simulink model "robot_v3_m1"  (R2022b)
settings: Solver=FixedStepDiscrete  StartTime=0.0  StopTime=10.0  FixedStep=T_S  RelTol=1e-3  EnableMultiTasking=on
values from neighbouring files (symbols this model uses):
  T_S = 10e-3    (= 0.01)    [robot_prototype_init.m]
undefined symbols (not defined in the file or in its folder): Break, Btn, btn, Button, Ctr, State, Up
libraries: legoev3lib x23
settings Model: ExtModeTrigDuration=2  Creator=hp  LastModifiedBy=hp
settings SolverCC: PositivePriorityOrder=on
settings OptimizationCC: EnhancedBackFolding=on  PassReuseOutputArgsAs=Individual arguments  ZeroExternalMemoryAtStartup=off  ZeroInternalMemoryAtStartup=off  MaxStackSize=64  OptimizeBlockOrder=speed  DifferentSizesBufferReuse=on  OptimizationCustomize=off  EfficientTunableParamExpr=on
settings DebuggingCC: ParameterTunabilityLossMsg=error
settings HardwareCC: ProdBitPerPointer=32  ProdBitPerSizeT=32  ProdBitPerPtrDiffT=32  ProdLargestAtomicInteger=Long  ProdWordSize=32  ProdHWDeviceType=ARM Compatible->ARM 9
settings SFSimCC: MATLABDynamicMemAlloc=off
settings RTWCC: Description=Embedded Coder  SystemTargetFile=ert.tlc  HardwareBoard=LEGO MINDSTORMS EV3  TLCOptions="-aInlineSetEventsForThisBaseRateFcn=TLC_FALSE -aSuppressMultiTaskScheduler=TLC_FALSE  -aRateBasedStepFcn=0"  TemplateMakefile=ert_default_tmf  Toolchain=Sourcery G++ Lite v2009q3
settings CodeAppCC: ForceParamTrailComments=on  IgnoreCustomStorageClasses=off  OperatorAnnotations=on  SimulinkDataObjDesc=on  SFDataObjDesc=on  InsertBlockDesc=on
settings ERTTargetCC: SupportContinuousTime=on  SupportVariableSizeSignals=on  ExtModeTransport=2  ExtModeStaticAlloc=on  ExtModeMexFile=ext_xcp  ExtModeIntrfLevel=Level2 - Open

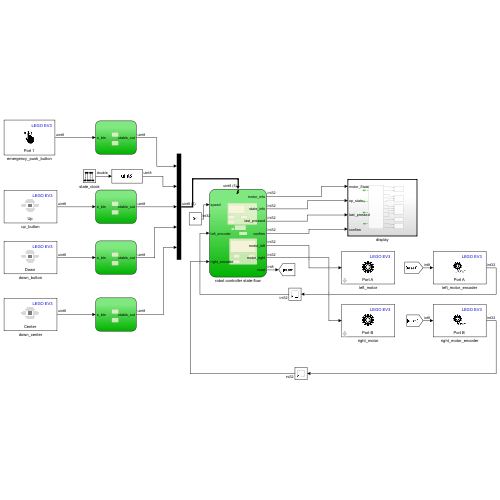
[thumbnail: Simulink's stored preview of the top-level diagram]
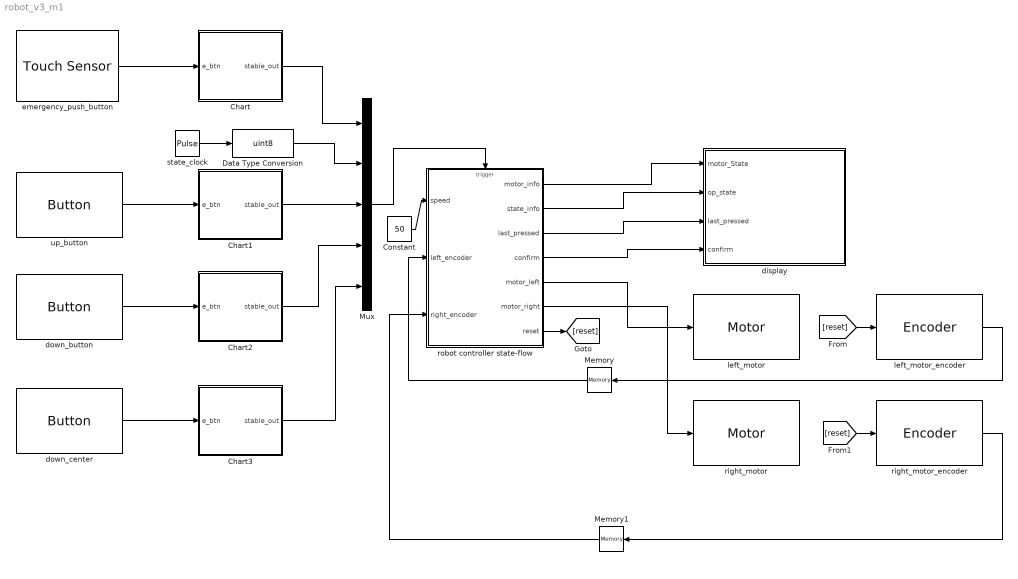
== system robot_v3_m1 ==
  Chart : Stateflow chart  TreatAsAtomicUnit=on
  Chart1 : Stateflow chart  TreatAsAtomicUnit=on
  Chart2 : Stateflow chart  TreatAsAtomicUnit=on
  Chart3 : Stateflow chart  TreatAsAtomicUnit=on
  Constant : Constant  Value=50  OutDataTypeStr=int32
  Data Type Conversion : DataTypeConversion  OutMin=0  OutMax=255  OutDataTypeStr=uint8  SaturateOnIntegerOverflow=off  RndMeth=Floor
  Memory : Memory
  Memory1 : Memory
  Mux : Mux  Inputs=5
  display : Subsystem  TreatAsAtomicUnit=on
  down_button : legoev3lib/Button  buttonType=Down  sampleTime=T_S
  down_center : legoev3lib/Button  buttonType=Center  sampleTime=T_S
  emergency_push_button : legoev3lib/Touch Sensor  portNumber=1  sampleTime=T_S
  left_motor : legoev3lib/Motor  sportNumber=A  sstopAction=Brake
  left_motor_encoder : legoev3lib/Encoder  portNumber=A  opMode=Reset by external signal  sampleTime=T_S
  right_motor : legoev3lib/Motor  sportNumber=B  sstopAction=Brake
  right_motor_encoder : legoev3lib/Encoder  portNumber=B  opMode=Reset by external signal  sampleTime=T_S
  robot controller state-flow : Stateflow chart  TreatAsAtomicUnit=on
  state_clock : DiscretePulseGenerator  Period=50  PulseWidth=25  PhaseDelay=20  SampleTime=T_S
  up_button : legoev3lib/Button  buttonType=Up  sampleTime=T_S
  wires:
  emergency_push_button/1 -> Chart/1(e_btn)
  robot controller state-flow/2(state_info) -> display/2(op_state)
  robot controller state-flow/1(motor_info) -> display/1(motor_State)
  Chart1/1(stable_out) -> Mux/3
  robot controller state-flow/4(confirm) -> display/4(confirm)
  robot controller state-flow/3(last_pressed) -> display/3(last_pressed)
  Chart3/1(stable_out) -> Mux/5
  up_button/1 -> Chart1/1(e_btn)
  Chart/1(stable_out) -> Mux/1
  Data Type Conversion/1 -> Mux/2
  Mux/1 -> robot controller state-flow/Trigger
  state_clock/1 -> Data Type Conversion/1
  down_button/1 -> Chart2/1(e_btn)
  Constant/1 -> robot controller state-flow/1(speed)
  down_center/1 -> Chart3/1(e_btn)
  Chart2/1(stable_out) -> Mux/4
  [reset] -> left_motor_encoder/1
  [reset] -> right_motor_encoder/1
  robot controller state-flow/5(motor_left) -> left_motor/1
  robot controller state-flow/6(motor_right) -> right_motor/1
  robot controller state-flow/7(reset) -> [reset]
  left_motor_encoder/1 -> Memory/1
  right_motor_encoder/1 -> Memory1/1
  Memory/1 -> robot controller state-flow/2(left_encoder)
  Memory1/1 -> robot controller state-flow/3(right_encoder)

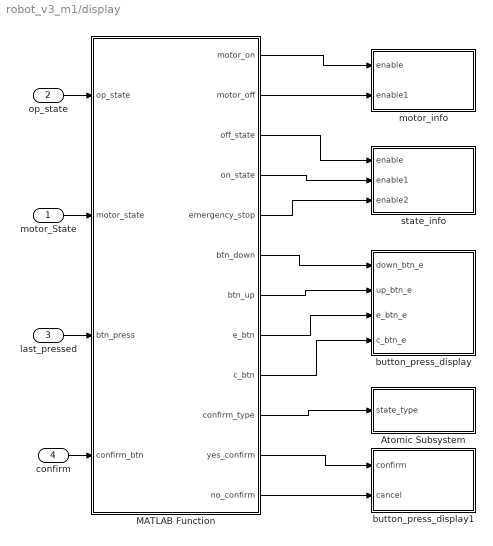
== system robot_v3_m1/display ==
  motor_State : Inport
  op_state : Inport  Port=2
  last_pressed : Inport  Port=3
  confirm : Inport  Port=4
  Atomic Subsystem : Subsystem
  MATLAB Function : MATLAB Function  TreatAsAtomicUnit=on
  button_press_display : Subsystem  SystemSampleTime=T_S
  button_press_display1 : Subsystem  SystemSampleTime=T_S
  motor_info : Subsystem  SystemSampleTime=T_S
  state_info : Subsystem  SystemSampleTime=T_S
  wires:
  op_state/1 -> MATLAB Function/1(op_state)
  motor_State/1 -> MATLAB Function/2(motor_state)
  MATLAB Function/3(off_state) -> state_info/1(enable)
  MATLAB Function/4(on_state) -> state_info/2(enable1)
  MATLAB Function/5(emergency_stop) -> state_info/3(enable2)
  MATLAB Function/1(motor_on) -> motor_info/1(enable)
  MATLAB Function/2(motor_off) -> motor_info/2(enable1)
  last_pressed/1 -> MATLAB Function/3(btn_press)
  MATLAB Function/6(btn_down) -> button_press_display/1(down_btn_e)
  MATLAB Function/7(btn_up) -> button_press_display/2(up_btn_e)
  MATLAB Function/8(e_btn) -> button_press_display/3(e_btn_e)
  confirm/1 -> MATLAB Function/4(confirm_btn)
  MATLAB Function/10(confirm_type) -> Atomic Subsystem/1(state_type)
  MATLAB Function/11(yes_confirm) -> button_press_display1/1(confirm)
  MATLAB Function/12(no_confirm) -> button_press_display1/2(cancel)
  MATLAB Function/9(c_btn) -> button_press_display/4(c_btn_e)

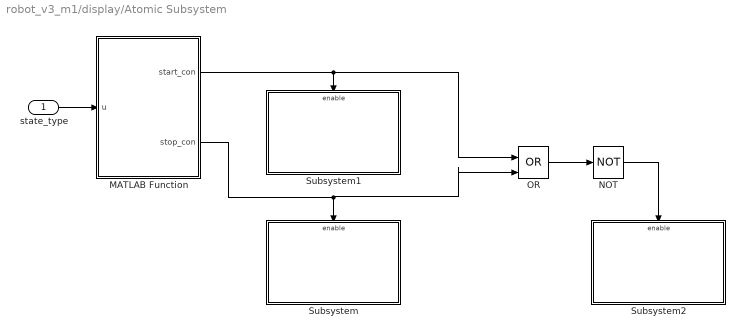
== system robot_v3_m1/display/Atomic Subsystem ==
  state_type : Inport
  MATLAB Function : MATLAB Function  TreatAsAtomicUnit=on
  NOT : Logic  Operator=NOT  IconShape=distinctive  AllPortsSameDT=off  OutDataTypeStr=boolean
  OR : Logic  Operator=OR  IconShape=distinctive  AllPortsSameDT=off  OutDataTypeStr=boolean
  Subsystem : Subsystem
  Subsystem1 : Subsystem
  Subsystem2 : Subsystem
  wires:
  state_type/1 -> MATLAB Function/1(u)
  MATLAB Function/1(start_con) -> OR/1, Subsystem1/Enable
  NOT/1 -> Subsystem2/Enable
  MATLAB Function/2(stop_con) -> OR/2, Subsystem/Enable
  OR/1 -> NOT/1

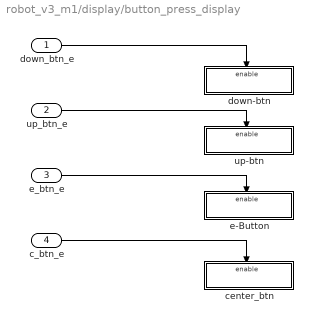
== system robot_v3_m1/display/button_press_display ==
  down_btn_e : Inport
  up_btn_e : Inport  Port=2
  e_btn_e : Inport  Port=3
  c_btn_e : Inport  Port=4
  center_btn : Subsystem
  down-btn : Subsystem
  e-Button : Subsystem
  up-btn : Subsystem
  wires:
  up_btn_e/1 -> up-btn/Enable
  down_btn_e/1 -> down-btn/Enable
  e_btn_e/1 -> e-Button/Enable
  c_btn_e/1 -> center_btn/Enable

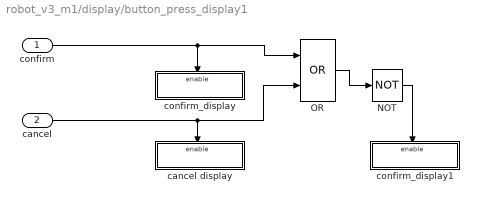
== system robot_v3_m1/display/button_press_display1 ==
  confirm : Inport
  cancel : Inport  Port=2
  NOT : Logic  Operator=NOT  IconShape=distinctive  AllPortsSameDT=off  OutDataTypeStr=boolean
  OR : Logic  Operator=OR  IconShape=distinctive  AllPortsSameDT=off  OutDataTypeStr=boolean
  cancel display : Subsystem
  confirm_display : Subsystem
  confirm_display1 : Subsystem
  wires:
  confirm/1 -> OR/1, confirm_display/Enable
  cancel/1 -> cancel display/Enable, OR/2
  OR/1 -> NOT/1
  NOT/1 -> confirm_display1/Enable

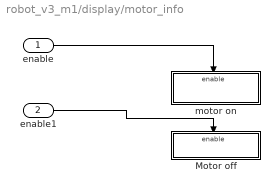
== system robot_v3_m1/display/motor_info ==
  enable : Inport
  enable1 : Inport  Port=2
  Motor off : Subsystem
  motor on : Subsystem
  wires:
  enable/1 -> motor on/Enable
  enable1/1 -> Motor off/Enable

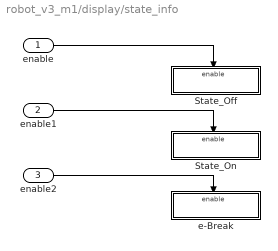
== system robot_v3_m1/display/state_info ==
  enable : Inport
  enable1 : Inport  Port=2
  enable2 : Inport  Port=3
  State_Off : Subsystem
  State_On : Subsystem
  e-Break : Subsystem
  wires:
  enable/1 -> State_Off/Enable
  enable2/1 -> e-Break/Enable
  enable1/1 -> State_On/Enable

== system robot_v3_m1/display/Atomic Subsystem/Subsystem ==
  Enable : EnablePort  StatesWhenEnabling=reset
  stop_confirm : legoev3lib/Display  slcdStr=STOP?  slcdLine=4  slcdFormat=Decimal

== system robot_v3_m1/display/Atomic Subsystem/Subsystem1 ==
  Enable : EnablePort  StatesWhenEnabling=reset
  start_confirm : legoev3lib/Display  slcdStr=START?  slcdLine=4  slcdFormat=Decimal

== system robot_v3_m1/display/Atomic Subsystem/Subsystem2 ==
  Enable : EnablePort  StatesWhenEnabling=reset
  start_confirm : legoev3lib/Display  slcdStr=>>  slcdLine=4  slcdFormat=Decimal

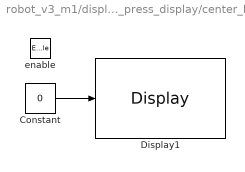
== system robot_v3_m1/display/button_press_display/center_btn ==
  enable : EnablePort  StatesWhenEnabling=reset
  Constant : Constant  Value=0
  Display1 : legoev3lib/Display  slcdStr=Ctr-Btn  slcdLine=10  slcdFormat=Hex
  wires:
  Constant/1 -> Display1/1

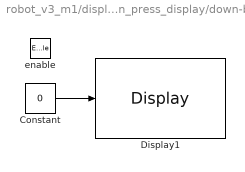
== system robot_v3_m1/display/button_press_display/down-btn ==
  enable : EnablePort  StatesWhenEnabling=reset
  Constant : Constant  Value=0
  Display1 : legoev3lib/Display  slcdStr=btn-down  slcdLine=10  slcdFormat=Hex
  wires:
  Constant/1 -> Display1/1

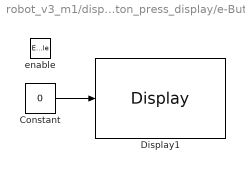
== system robot_v3_m1/display/button_press_display/e-Button ==
  enable : EnablePort  StatesWhenEnabling=reset
  Constant : Constant  Value=0
  Display1 : legoev3lib/Display  slcdStr=E-Button  slcdLine=10  slcdFormat=Hex
  wires:
  Constant/1 -> Display1/1

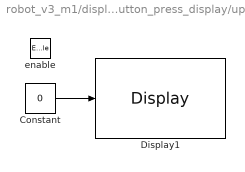
== system robot_v3_m1/display/button_press_display/up-btn ==
  enable : EnablePort  StatesWhenEnabling=reset
  Constant : Constant  Value=0
  Display1 : legoev3lib/Display  slcdStr=btn-Up  slcdLine=10  slcdFormat=Hex
  wires:
  Constant/1 -> Display1/1

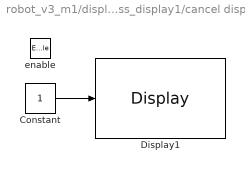
== system robot_v3_m1/display/button_press_display1/cancel display ==
  enable : EnablePort  StatesWhenEnabling=reset
  Constant : Constant
  Display1 : legoev3lib/Display  slcdStr=Cancel  slcdLine=5  slcdFormat=Hex
  wires:
  Constant/1 -> Display1/1

== system robot_v3_m1/display/button_press_display1/confirm_display ==
  enable : EnablePort  StatesWhenEnabling=reset
  Constant : Constant
  Display1 : legoev3lib/Display  slcdStr=Confrim  slcdLine=5  slcdFormat=Hex
  wires:
  Constant/1 -> Display1/1

== system robot_v3_m1/display/button_press_display1/confirm_display1 ==
  enable : EnablePort  StatesWhenEnabling=reset
  Display1 : legoev3lib/Display  slcdStr=>>  slcdLine=5  slcdFormat=Hex

== system robot_v3_m1/display/motor_info/Motor off ==
  enable : EnablePort  StatesWhenEnabling=reset
  Constant : Constant  Value=0
  Display1 : legoev3lib/Display  slcdStr=motorOff  slcdLine=2  slcdFormat=Hex
  wires:
  Constant/1 -> Display1/1

== system robot_v3_m1/display/motor_info/motor on ==
  enable : EnablePort  StatesWhenEnabling=reset
  Constant : Constant  Value=0  SampleTime=T_S
  Display1 : legoev3lib/Display  slcdStr=motorOn  slcdLine=2  slcdFormat=Hex
  wires:
  Constant/1 -> Display1/1

== system robot_v3_m1/display/state_info/State_Off ==
  enable : EnablePort  StatesWhenEnabling=reset
  Constant : Constant  Value=0
  Display1 : legoev3lib/Display  slcdStr=StateOff  slcdLine=1  slcdFormat=Hex
  wires:
  Constant/1 -> Display1/1

== system robot_v3_m1/display/state_info/State_On ==
  enable : EnablePort  StatesWhenEnabling=reset
  Constant : Constant  Value=0
  Display1 : legoev3lib/Display  slcdStr=State-On  slcdLine=1  slcdFormat=Hex
  wires:
  Constant/1 -> Display1/1

== system robot_v3_m1/display/state_info/e-Break ==
  enable : EnablePort  StatesWhenEnabling=reset
  Constant : Constant  Value=0
  Display1 : legoev3lib/Display  slcdStr=E-Break  slcdLine=1  slcdFormat=Hex
  wires:
  Constant/1 -> Display1/1

== stateflow chart robot_v3_m1/Chart ==
  state off
    entry:
    stable_out = 0
  note: ]
  state on
    entry:
    stable_out = 1
  (default) -> off
  on -> off : [duration(e_btn<0.3) > 20e-3]
  off -> on : [duration(e_btn> 0.7) > 20e-3]
  data: e_btn input; stable_out output uint8

== matlab function robot_v3_m1/display/MATLAB Function ==
  data: op_state input; motor_on output; motor_off output; motor_state input; off_state output; on_state output; emergency_stop output; btn_down output; btn_up output; e_btn output; c_btn output; btn_press input; confirm_btn input; confirm_type output; yes_confirm output; no_confirm output
function [motor_on,motor_off, off_state, on_state, emergency_stop, btn_down, btn_up ,e_btn, c_btn , confirm_type ,yes_confirm, no_confirm] = fcn(op_state, motor_state, btn_press, confirm_btn)

motor_on = 0;
motor_off = 0;

off_state = 0;
on_state = 0;
emergency_stop = 0;

btn_down = 0;
btn_up = 0;
e_btn = 0;
c_btn = 0;

confirm_type = 0;
yes_confirm = 0;
no_confirm = 0;

% for displaying motor state
if motor_state == 0
    motor_off = 1;
elseif motor_state == 1
    motor_on = 1;
end

% for displaying states
if op_state == 0
    off_state = 1;
elseif op_state == 1
    on_state = 1;
elseif op_state == 2
    emergency_stop = 1;
end

%for displaying button press
if btn_press == 1
    btn_down = 1;
elseif btn_press == 2
    btn_up = 1;
elseif btn_press == 3
    e_btn = 1;
elseif btn_press == 4
    c_btn = 1;
end

%for displaying which action to confirm
%i.e. either star action or stop action
if confirm_btn == 1 | confirm_btn == 2
    confirm_type = 1;
elseif confirm_btn == 3 | confirm_btn == 4
    confirm_type = 2;
end

if confirm_btn == 1 && confirm_type == 1
    yes_confirm = 1;
elseif confirm_btn == 2 && confirm_type == 1
    no_confirm = 1;
end

if confirm_btn == 3 && confirm_type == 2
    yes_confirm = 1;
elseif confirm_btn == 4 && confirm_type == 2
    no_confirm = 1;
end

== stateflow chart robot_v3_m1/robot controller state-flow ==
  state Off_super_state
    entry:
    state state_off
      entry:
      motor_left = 0;
      motor_right = 0;
      motor_info = 0;
      state_info = 0;
      confirm = 0;
      e_press_count = 0;
      last_pressed = button_type;
      stop_robot = int32(0);
    state confirm_start_action_
      entry:
      confirm = 1;
      last_pressed = button_type;
    state cancel_start_action
      entry:
      confirm = 2;
      last_pressed = button_type;
    state confirmed_start
      entry:
      start_robot = 1;
      last_pressed = button_type;
      confirm = 0;
    (default) -> state_off
    state_off -> confirm_start_action_ : up_btn{button_type = 2}
    cancel_start_action -> state_off [order 1] : center_btn{confirm = 0;
        | button_type = 4;}
    cancel_start_action -> confirm_start_action_ [order 2] : up_btn{button_type = 2;}
    confirm_start_action_ -> cancel_start_action [order 2] : down_btn{button_type = 1}
    confirm_start_action_ -> confirmed_start [order 1] : center_btn{
        | button_type = 4}
  note: button_type is internal variable used to store which button was pressed
      | 0 = no button press
      | 1 = down
      | 2 = up
      | 3 = emergency_button
      | 4 = center_button
  note: These confirmation applies when confirming to turn on the robot
      |
      | confirm = 1
      | display 1 at the confirm position
      | confirm = 2
      | display 1 at cancel position
      |
      | 0
      | anything else don't display anything.
  state emergency_stop
    entry:
    motor_left = 0;
    motor_right = 0;
    motor_info = 0;
    state_info = 2;
    last_pressed = button_type;
  note: state_info
      | 0 = off_state
      | 1 = Turned on
      | 2 = emergency top
  state leyway
    entry:
    reset = 0;
  state intermediate
    entry:
    e_press_count = e_press_count +1;
  state go
    entry:
    state action
      entry:
      motor_info = 1;
      state_info = 1;
      last_pressed = button_type;
      start_robot = int32(0);
      e_press_count = int32(0);
      during:
      if (2046 - left_encoder) >0
      motor_left  =  speed;
      else
      motor_left = 0;
      end
      if (2046 - right_encoder) >0
      motor_right  =  speed;
      else
      motor_right = 0;
      end
      exit:
      motor_left = 0;
      motor_right = 0;
    state confirm_stop_action
      entry:
      confirm = 3;
      motor_info = 0;
      last_pressed = button_type;
    state cancel_stop_action
      entry:
      confirm = 4;
      last_pressed = button_type;
    state confirmed_stop
      entry:
      stop_robot = 1;
      last_pressed = button_type;
      confirm = 0;
      exit:
      reset = 1;
    (default) -> action
    action -> confirm_stop_action : down_btn{button_type = 1}
    cancel_stop_action -> action [order 1] : center_btn{confirm = 0;
        | button_type = 4;}
    cancel_stop_action -> confirm_stop_action [order 2] : up_btn{button_type = 2;}
    confirm_stop_action -> cancel_stop_action [order 2] : down_btn{button_type = 1}
    confirm_stop_action -> confirmed_stop [order 1] : center_btn{
        | button_type = 4}
  (default) -> Off_super_state
  go -> Off_super_state [order 2] : [stop_robot == 1]{confirm = 0; button_type = 1;}
  Off_super_state -> leyway : [start_robot == 1]{button_type = 4;confirm = 0;}
  go -> emergency_stop [order 1] : emergency_btn{
      | button_type = 3}
  emergency_stop -> go [order 2] : [e_press_count == 2]
  emergency_stop -> intermediate [order 1] : emergency_btn
  intermediate -> emergency_stop [order 1] : after(0.5, sec){e_press_count = 0;}
  intermediate -> emergency_stop [order 2] : emergency_btn{e_press_count = e_press_count+1;}
  leyway -> go : after(5, sec)
  data: speed input int32; motor_info output int32; state_info output int32; button_type local int32 =int32(0); last_pressed output int32; confirm output int32; start_robot local int32 =int32(0); e_press_count local int32 =int32(0); motor_left output int32; motor_right output int32; reset output int8; left_encoder input int32; right_encoder input int32; stop_robot local int32
  events: emergency_btn input RISING_EDGE_EVENT; active_chart input RISING_EDGE_EVENT; up_btn input RISING_EDGE_EVENT; down_btn input RISING_EDGE_EVENT; center_btn input RISING_EDGE_EVENT

== matlab function robot_v3_m1/display/Atomic Subsystem/MATLAB Function ==
  data: u input; start_con output; stop_con output
function [start_con, stop_con]= fcn(u)

start_con = 0;
stop_con = 0;

if u == 1
    start_con = 1;
elseif u == 2
    stop_con = 1;
end

== stateflow chart robot_v3_m1/Chart1 ==
  state off
    entry:
    stable_out = 0
  note: ]
  state on
    entry:
    stable_out = 1
  (default) -> off
  on -> off : [duration(e_btn<0.3) > 20e-3]
  off -> on : [duration(e_btn> 0.7) > 20e-3]
  data: e_btn input; stable_out output uint8

== stateflow chart robot_v3_m1/Chart2 ==
  state off
    entry:
    stable_out = 0
  note: ]
  state on
    entry:
    stable_out = 1
  (default) -> off
  on -> off : [duration(e_btn<0.3) > 20e-3]
  off -> on : [duration(e_btn> 0.7) > 20e-3]
  data: e_btn input; stable_out output uint8

== stateflow chart robot_v3_m1/Chart3 ==
  state off
    entry:
    stable_out = 0
  note: ]
  state on
    entry:
    stable_out = 1
  (default) -> off
  on -> off : [duration(e_btn<0.3) > 20e-3]
  off -> on : [duration(e_btn> 0.7) > 20e-3]
  data: e_btn input; stable_out output uint8
